simulink model "stopWatch"  (R2018a)
settings: Solver=VariableStepAuto  StartTime=0.0  StopTime=0.2  RelTol=1e-3
libraries: simulink_extras x1
settings Model: Creator=86188  LastModifiedBy=86188

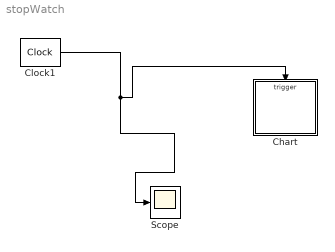
== system stopWatch ==
  Chart : Stateflow chart  TreatAsAtomicUnit=on
  Clock1 : simulink_extras/Flip Flops/Clock  period=0.2
  Scope : Scope
  wires:
  Clock1/1 -> Scope/1, Chart/Trigger

== stateflow chart stopWatch/Chart ==
  settings: executeAtInitialization=1
  state StopW
    en:f("en_StopW");
    state Reset
      en:f("en_Reset");send(LAP);send(START);
      Reset -> (junction 7) [order 1] : LAP{cent=0;sec=0;mins=0;
          | disp_cent=0;disp_sec=0;
          | disp_min=0;}
    state LapStop
      en:f("en_LapStop");
    (default) -> Reset
    LapStop -> Reset [order 1] : LAP
  state RunW
    en:f("en_RunW");
    state Running
      du:
      f("edu_Running");
      disp_cent=cent;
      disp_sec=sec;
      disp_min=mins;
    state Lap
      en:f("Lap");
    RunW -> (junction 26) : TIC{f("cond_TIC");cent=cent+1;}
    (junction 26) -> (junction 28) [order 1] : [cent==100]{cent=0;sec=sec+1;}
    (junction 26) -> (junction 30) [order 2]
    (junction 28) -> (junction 30) [order 2]
    (junction 28) -> (junction 30) [order 1] : [sec==60]{sec=0;mins=mins+1;}
    Running -> Lap [order 1] : LAP
    Lap -> Running [order 1] : LAP
  (default) -> StopW
  Reset -> Running [order 1] : START
  Running -> Reset [order 2] : START
  LapStop -> Lap [order 2] : START
  Lap -> LapStop [order 2] : START
  data: s function_input; cent local double =0; sec local double =0; mins local double =0; disp_cent local double =0; disp_sec local double =0; disp_min local double =0
  events: LAP local FUNCTION_CALL_EVENT; START local FUNCTION_CALL_EVENT; TIC input EITHER_EDGE_EVENT
  function f(s):
    | function f(s)
    |   fprintf(s+' %.3f %.3f\n', cent, sec);
